simulink model "PTEngineCU"  (Simulink 10.1)
settings: Solver=ode45  StartTime=0.0  StopTime=inf  RelTol=1e-3  EnableMultiTasking=on
PreLoadFcn:
  | Trq_x = [500.0, 600.0, 700.0, 800.0, 1000.0, 2000.0, 3000.0, 4000.0, 4500.0, 5000.0, 6000.0, 7000.0, 8000.0];
  | TrqFull_y = [10.0, 40.0, 70.0, 95.0, 120.0, 145.0, 165.0, 180.0, 185.0, 182.0, 168.0, 130.0, 0.0];
  | 
  | TrqDrag_y = [-10.0, -10.0, -10.0, -10.0, -10.0, -20.0, -30.0, -40.0, -45.0, -50.0, -60.0, -70.0, -80.0];
  | 
  | TrqOpt_y = [0.0, 0.0, 0.0, 0.0, 0.0, 0.0, 0.0, 0.0, 0.0, 0.0, 0.0, 0.0, 0.0];
InitFcn:
  | Trq_x = [500.0, 600.0, 700.0, 800.0, 1000.0, 2000.0, 3000.0, 4000.0, 4500.0, 5000.0, 6000.0, 7000.0, 8000.0];
  | TrqFull_y = [10.0, 40.0, 70.0, 95.0, 120.0, 145.0, 165.0, 180.0, 185.0, 182.0, 168.0, 130.0, 0.0];
  | 
  | TrqDrag_y = [-10.0, -10.0, -10.0, -10.0, -10.0, -20.0, -30.0, -40.0, -45.0, -50.0, -60.0, -70.0, -80.0];
  | 
  | TrqOpt_y = [0.0, 0.0, 0.0, 0.0, 0.0, 0.0, 0.0, 0.0, 0.0, 0.0, 0.0, 0.0, 0.0];
libraries: simulink x7, CarMaker4SL x4
(part 2 of 2)

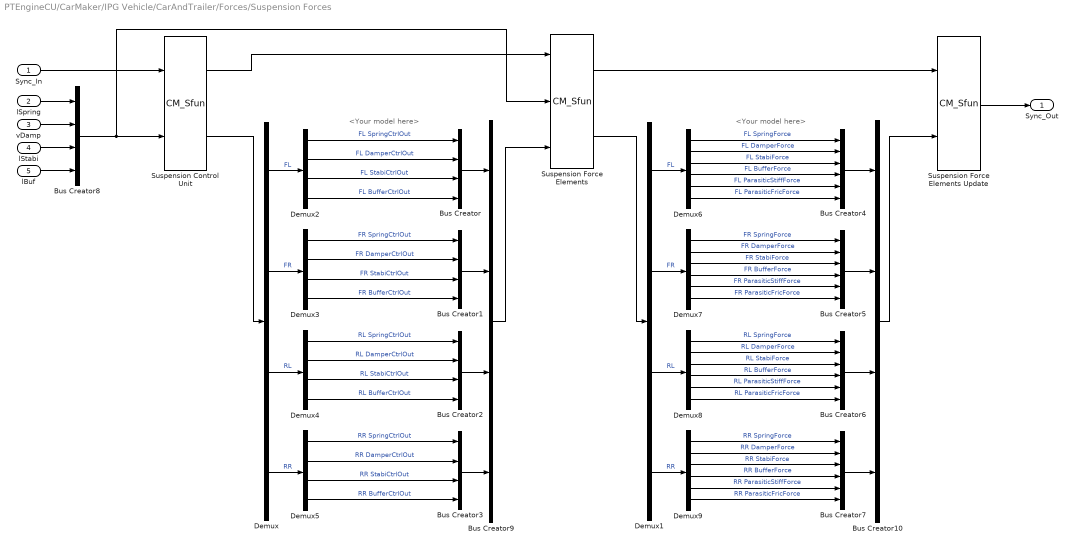
== system PTEngineCU/CarMaker/IPG Vehicle/CarAndTrailer/Forces/Suspension Forces ==
  note: <Your model here>
  note: <Your model here>
  Sync_In : Inport
  lSpring : Inport  Port=2
  vDamp : Inport  Port=3
  lStabi : Inport  Port=4
  lBuf : Inport  Port=5
  Bus Creator{,1..3,8..10} (7 alike) : BusCreator  Inputs=4
  Bus Creator{4..7} (4 alike) : BusCreator  Inputs=6
  Demux{,1..5} (6 alike) : Demux
  Demux{6..9} (4 alike) : Demux  Outputs=6
  Suspension Control Unit : S-Function  FunctionName=CM_Sfun  Parameters='ForcesSuspControl'  SFunctionDeploymentMode=off  EnableBusSupport=off
  Suspension Force Elements : S-Function  FunctionName=CM_Sfun  Parameters='ForcesSusp'  SFunctionDeploymentMode=off  EnableBusSupport=off
  Suspension Force Elements Update : S-Function  FunctionName=CM_Sfun  Parameters='ForcesSuspUpd'  SFunctionDeploymentMode=off  EnableBusSupport=off
  Sync_Out : Outport  VectorParamsAs1DForOutWhenUnconnected=off
  wires:
  vDamp/1 -> Bus Creator8/2
  lStabi/1 -> Bus Creator8/3
  lBuf/1 -> Bus Creator8/4
  lSpring/1 -> Bus Creator8/1
  Bus Creator8/1 -> Suspension Control Unit/2, Suspension Force Elements/2
  Sync_In/1 -> Suspension Control Unit/1
  Suspension Control Unit/1 -> Suspension Force Elements/1
  Suspension Force Elements/1 -> Suspension Force Elements Update/1
  Suspension Force Elements Update/1 -> Sync_Out/1
  Bus Creator4/1 -> Bus Creator10/1
  Bus Creator5/1 -> Bus Creator10/2
  Bus Creator6/1 -> Bus Creator10/3
  Bus Creator7/1 -> Bus Creator10/4
  Demux6/1 -> Bus Creator4/1  "FL SpringForce"
  Demux9/1 -> Bus Creator7/1  "RR SpringForce"
  Demux9/2 -> Bus Creator7/2  "RR DamperForce"
  Demux9/3 -> Bus Creator7/3  "RR StabiForce"
  Demux9/4 -> Bus Creator7/4  "RR BufferForce"
  Demux9/5 -> Bus Creator7/5  "RR ParasiticStiffForce"
  Demux9/6 -> Bus Creator7/6  "RR ParasiticFricForce"
  Demux8/1 -> Bus Creator6/1  "RL SpringForce"
  Demux8/2 -> Bus Creator6/2  "RL DamperForce"
  Demux8/4 -> Bus Creator6/4  "RL BufferForce"
  Demux8/5 -> Bus Creator6/5  "RL ParasiticStiffForce"
  Demux8/6 -> Bus Creator6/6  "RL ParasiticFricForce"
  Demux8/3 -> Bus Creator6/3  "RL StabiForce"
  Demux7/1 -> Bus Creator5/1  "FR SpringForce"
  Demux7/2 -> Bus Creator5/2  "FR DamperForce"
  Demux7/3 -> Bus Creator5/3  "FR StabiForce"
  Demux7/4 -> Bus Creator5/4  "FR BufferForce"
  Demux7/5 -> Bus Creator5/5  "FR ParasiticStiffForce"
  Demux7/6 -> Bus Creator5/6  "FR ParasiticFricForce"
  Demux6/2 -> Bus Creator4/2  "FL DamperForce"
  Demux6/3 -> Bus Creator4/3  "FL StabiForce"
  Demux6/4 -> Bus Creator4/4  "FL BufferForce"
  Demux6/5 -> Bus Creator4/5  "FL ParasiticStiffForce"
  Demux6/6 -> Bus Creator4/6  "FL ParasiticFricForce"
  Bus Creator10/1 -> Suspension Force Elements Update/2
  Demux/1 -> Demux2/1  "FL"
  Bus Creator1/1 -> Bus Creator9/2
  Demux/2 -> Demux3/1  "FR"
  Bus Creator2/1 -> Bus Creator9/3
  Demux/3 -> Demux4/1  "RL"
  Bus Creator3/1 -> Bus Creator9/4
  Demux2/1 -> Bus Creator/1  "FL SpringCtrlOut"
  Demux/4 -> Demux5/1  "RR"
  Demux5/1 -> Bus Creator3/1  "RR SpringCtrlOut"
  Demux5/2 -> Bus Creator3/2  "RR DamperCtrlOut"
  Demux5/3 -> Bus Creator3/3  "RR StabiCtrlOut"
  Demux5/4 -> Bus Creator3/4  "RR BufferCtrlOut"
  Demux4/1 -> Bus Creator2/1  "RL SpringCtrlOut"
  Demux4/2 -> Bus Creator2/2  "RL DamperCtrlOut"
  Demux4/4 -> Bus Creator2/4  "RL BufferCtrlOut"
  Demux4/3 -> Bus Creator2/3  "RL StabiCtrlOut"
  Demux3/1 -> Bus Creator1/1  "FR SpringCtrlOut"
  Demux3/2 -> Bus Creator1/2  "FR DamperCtrlOut"
  Demux3/3 -> Bus Creator1/3  "FR StabiCtrlOut"
  Demux3/4 -> Bus Creator1/4  "FR BufferCtrlOut"
  Demux2/2 -> Bus Creator/2  "FL DamperCtrlOut"
  Demux2/3 -> Bus Creator/3  "FL StabiCtrlOut"
  Demux2/4 -> Bus Creator/4  "FL BufferCtrlOut"
  Suspension Control Unit/2 -> Demux/1
  Bus Creator9/1 -> Suspension Force Elements/3
  Bus Creator/1 -> Bus Creator9/1
  Suspension Force Elements/2 -> Demux1/1
  Demux1/1 -> Demux6/1  "FL"
  Demux1/2 -> Demux7/1  "FR"
  Demux1/3 -> Demux8/1  "RL"
  Demux1/4 -> Demux9/1  "RR"

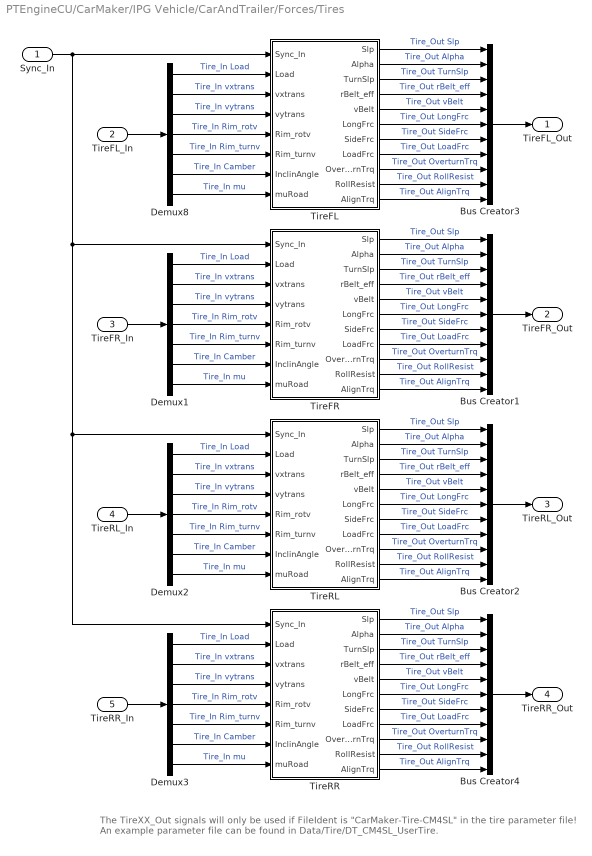
== system PTEngineCU/CarMaker/IPG Vehicle/CarAndTrailer/Forces/Tires ==
  note: The TireXX_Out signals will only be used if FileIdent is "CarMaker-Tire-CM4SL" in the tire parameter file!
      | An example parameter file can be found in Data/Tire/DT_CM4SL_UserTire.
  Sync_In : Inport
  TireFL_In : Inport  Port=2
  TireFR_In : Inport  Port=3
  TireRL_In : Inport  Port=4
  TireRR_In : Inport  Port=5
  Bus Creator{1..4} (4 alike) : BusCreator  Inputs=11
  Demux{1..3,8} (4 alike) : Demux  Outputs=7
      settings: DisplayOption=none
  TireFL : Subsystem
  TireFR : Subsystem
  TireRL : Subsystem
  TireRR : Subsystem
  TireFL_Out : Outport  VectorParamsAs1DForOutWhenUnconnected=off
  TireFR_Out : Outport  Port=2  VectorParamsAs1DForOutWhenUnconnected=off
  TireRL_Out : Outport  Port=3  VectorParamsAs1DForOutWhenUnconnected=off
  TireRR_Out : Outport  Port=4  VectorParamsAs1DForOutWhenUnconnected=off
  wires:
  Sync_In/1 -> TireRR/1(Sync_In), TireRL/1(Sync_In), TireFR/1(Sync_In), TireFL/1(Sync_In)
  Bus Creator4/1 -> TireRR_Out/1
  Bus Creator2/1 -> TireRL_Out/1
  Bus Creator1/1 -> TireFR_Out/1
  Demux3/5 -> TireRR/6(Rim_turnv)  "Tire_In Rim_turnv"
  Demux3/4 -> TireRR/5(Rim_rotv)  "Tire_In Rim_rotv"
  Demux3/1 -> TireRR/2(Load)  "Tire_In Load"
  Demux3/7 -> TireRR/8(muRoad)  "Tire_In mu"
  Demux3/6 -> TireRR/7(InclinAngle)  "Tire_In Camber"
  Demux3/2 -> TireRR/3(vxtrans)  "Tire_In vxtrans"
  Demux3/3 -> TireRR/4(vytrans)  "Tire_In vytrans"
  TireRR/11(AlignTrq) -> Bus Creator4/11  "Tire_Out AlignTrq"
  TireRR/10(RollResist) -> Bus Creator4/10  "Tire_Out RollResist"
  TireRR/9(OverturnTrq) -> Bus Creator4/9  "Tire_Out OverturnTrq"
  TireRR/8(LoadFrc) -> Bus Creator4/8  "Tire_Out LoadFrc"
  TireRR/7(SideFrc) -> Bus Creator4/7  "Tire_Out SideFrc"
  TireRR/6(LongFrc) -> Bus Creator4/6  "Tire_Out LongFrc"
  TireRR/5(vBelt) -> Bus Creator4/5  "Tire_Out vBelt"
  TireRR/4(rBelt_eff) -> Bus Creator4/4  "Tire_Out rBelt_eff"
  TireRR/3(TurnSlp) -> Bus Creator4/3  "Tire_Out TurnSlp"
  TireRR/1(Slp) -> Bus Creator4/1  "Tire_Out Slp"
  TireRR/2(Alpha) -> Bus Creator4/2  "Tire_Out Alpha"
  Demux2/5 -> TireRL/6(Rim_turnv)  "Tire_In Rim_turnv"
  Demux2/4 -> TireRL/5(Rim_rotv)  "Tire_In Rim_rotv"
  Demux2/1 -> TireRL/2(Load)  "Tire_In Load"
  Demux2/7 -> TireRL/8(muRoad)  "Tire_In mu"
  Demux2/6 -> TireRL/7(InclinAngle)  "Tire_In Camber"
  Demux2/2 -> TireRL/3(vxtrans)  "Tire_In vxtrans"
  Demux2/3 -> TireRL/4(vytrans)  "Tire_In vytrans"
  TireRL/11(AlignTrq) -> Bus Creator2/11  "Tire_Out AlignTrq"
  TireRL/10(RollResist) -> Bus Creator2/10  "Tire_Out RollResist"
  TireRL/9(OverturnTrq) -> Bus Creator2/9  "Tire_Out OverturnTrq"
  TireRL/8(LoadFrc) -> Bus Creator2/8  "Tire_Out LoadFrc"
  TireRL/7(SideFrc) -> Bus Creator2/7  "Tire_Out SideFrc"
  TireRL/6(LongFrc) -> Bus Creator2/6  "Tire_Out LongFrc"
  TireRL/5(vBelt) -> Bus Creator2/5  "Tire_Out vBelt"
  TireRL/4(rBelt_eff) -> Bus Creator2/4  "Tire_Out rBelt_eff"
  TireRL/3(TurnSlp) -> Bus Creator2/3  "Tire_Out TurnSlp"
  TireRL/1(Slp) -> Bus Creator2/1  "Tire_Out Slp"
  TireRL/2(Alpha) -> Bus Creator2/2  "Tire_Out Alpha"
  Demux1/5 -> TireFR/6(Rim_turnv)  "Tire_In Rim_turnv"
  Demux1/4 -> TireFR/5(Rim_rotv)  "Tire_In Rim_rotv"
  Demux1/1 -> TireFR/2(Load)  "Tire_In Load"
  Demux1/7 -> TireFR/8(muRoad)  "Tire_In mu"
  Demux1/6 -> TireFR/7(InclinAngle)  "Tire_In Camber"
  Demux1/2 -> TireFR/3(vxtrans)  "Tire_In vxtrans"
  Demux1/3 -> TireFR/4(vytrans)  "Tire_In vytrans"
  TireFR/11(AlignTrq) -> Bus Creator1/11  "Tire_Out AlignTrq"
  TireFR/10(RollResist) -> Bus Creator1/10  "Tire_Out RollResist"
  TireFR/9(OverturnTrq) -> Bus Creator1/9  "Tire_Out OverturnTrq"
  TireFR/8(LoadFrc) -> Bus Creator1/8  "Tire_Out LoadFrc"
  TireFR/7(SideFrc) -> Bus Creator1/7  "Tire_Out SideFrc"
  TireFR/6(LongFrc) -> Bus Creator1/6  "Tire_Out LongFrc"
  TireFR/5(vBelt) -> Bus Creator1/5  "Tire_Out vBelt"
  TireFR/4(rBelt_eff) -> Bus Creator1/4  "Tire_Out rBelt_eff"
  TireFR/3(TurnSlp) -> Bus Creator1/3  "Tire_Out TurnSlp"
  TireFR/1(Slp) -> Bus Creator1/1  "Tire_Out Slp"
  TireFR/2(Alpha) -> Bus Creator1/2  "Tire_Out Alpha"
  Demux8/5 -> TireFL/6(Rim_turnv)  "Tire_In Rim_turnv"
  Demux8/4 -> TireFL/5(Rim_rotv)  "Tire_In Rim_rotv"
  TireFL_In/1 -> Demux8/1
  Demux8/1 -> TireFL/2(Load)  "Tire_In Load"
  Demux8/7 -> TireFL/8(muRoad)  "Tire_In mu"
  Demux8/6 -> TireFL/7(InclinAngle)  "Tire_In Camber"
  Demux8/2 -> TireFL/3(vxtrans)  "Tire_In vxtrans"
  Demux8/3 -> TireFL/4(vytrans)  "Tire_In vytrans"
  TireFL/11(AlignTrq) -> Bus Creator3/11  "Tire_Out AlignTrq"
  TireFL/10(RollResist) -> Bus Creator3/10  "Tire_Out RollResist"
  TireFL/9(OverturnTrq) -> Bus Creator3/9  "Tire_Out OverturnTrq"
  TireFL/8(LoadFrc) -> Bus Creator3/8  "Tire_Out LoadFrc"
  TireFL/7(SideFrc) -> Bus Creator3/7  "Tire_Out SideFrc"
  TireFL/6(LongFrc) -> Bus Creator3/6  "Tire_Out LongFrc"
  TireFL/5(vBelt) -> Bus Creator3/5  "Tire_Out vBelt"
  TireFL/4(rBelt_eff) -> Bus Creator3/4  "Tire_Out rBelt_eff"
  TireFL/3(TurnSlp) -> Bus Creator3/3  "Tire_Out TurnSlp"
  TireFL/1(Slp) -> Bus Creator3/1  "Tire_Out Slp"
  TireFL/2(Alpha) -> Bus Creator3/2  "Tire_Out Alpha"
  Bus Creator3/1 -> TireFL_Out/1
  TireFR_In/1 -> Demux1/1
  TireRL_In/1 -> Demux2/1
  TireRR_In/1 -> Demux3/1

== system PTEngineCU/CarMaker/IPG Vehicle/CarAndTrailer/Forces/Vehicle Forces ==
  Sync_In : Inport
  Bus Creator1 : BusCreator  Inputs=12
  Bus Creator8 : BusCreator  Inputs=16
  BusCreator1 : BusCreator  Inputs=4
  BusCreator2 : BusCreator  Inputs=9
  Demux : Demux  Outputs=16
      settings: DisplayOption=none
  Demux1 : Demux  Outputs=12
      settings: DisplayOption=none
  Demux2 : Demux  Outputs=13
      settings: DisplayOption=none
  Forces : S-Function  FunctionName=CM_Sfun  Parameters='Forces'  SFunctionDeploymentMode=off  EnableBusSupport=off
  Terminator : Terminator
  Sync_Out : Outport  VectorParamsAs1DForOutWhenUnconnected=off
  Car.Virtual : Outport  Port=2  VectorParamsAs1DForOutWhenUnconnected=off
  Car.Aero : Outport  Port=3  VectorParamsAs1DForOutWhenUnconnected=off
  Car.Load : Outport  Port=4  VectorParamsAs1DForOutWhenUnconnected=off
  wires:
  BusCreator1/1 -> Terminator/1  "Aero IF (in)"
  Demux2/13 -> BusCreator2/9  "car Aero Trq_1 z"
  Demux2/12 -> BusCreator2/8  "car Aero Trq_1 y"
  Demux2/11 -> BusCreator2/7  "car Aero Trq_1 x"
  Demux2/10 -> BusCreator2/6  "car Aero Frc_1 z"
  Demux2/9 -> BusCreator2/5  "car Aero Frc_1 y"
  Demux2/8 -> BusCreator2/4  "car Aero Frc_1 x"
  Demux2/7 -> BusCreator2/3  "car Aero PoA_1 z"
  Demux2/6 -> BusCreator2/2  "car Aero PoA_1 y"
  Demux2/5 -> BusCreator2/1  "car Aero PoA_1 x"
  Demux2/4 -> BusCreator1/4  "car Aero tau_1"
  Demux2/3 -> BusCreator1/3  "car Aero ApproachVel_1 z"
  Demux2/2 -> BusCreator1/2  "car Aero ApproachVel_1 y"
  Demux2/1 -> BusCreator1/1  "car Aero ApproachVel_1 x"
  Demux/16 -> Bus Creator8/16  "Car Load_3 tz"
  Demux/15 -> Bus Creator8/15  "Car Load_3 ty"
  Demux/14 -> Bus Creator8/14  "Car Load_3 tx"
  Demux/13 -> Bus Creator8/13  "Car Load_3 mass"
  Demux1/12 -> Bus Creator1/12  "Car Virtual Trq_0 z"
  Demux1/11 -> Bus Creator1/11  "Car Virtual Trq_0 y"
  Demux1/10 -> Bus Creator1/10  "Car Virtual Trq_0 x"
  Demux1/9 -> Bus Creator1/9  "Car Virtual Trq_1 z"
  Demux1/8 -> Bus Creator1/8  "Car Virtual Trq_1 y"
  Demux1/7 -> Bus Creator1/7  "Car Virtual Trq_1 x"
  Demux1/6 -> Bus Creator1/6  "Car Virtual Frc_0 z"
  Demux1/5 -> Bus Creator1/5  "Car Virtual Frc_0 y"
  Demux1/4 -> Bus Creator1/4  "Car Virtual Frc_0 x"
  Sync_In/1 -> Forces/1
  Forces/1 -> Sync_Out/1
  BusCreator2/1 -> Car.Aero/1
  Demux1/1 -> Bus Creator1/1  "Car Virtual Frc_1 x"
  Demux1/2 -> Bus Creator1/2  "Car Virtual Frc_1 y"
  Demux1/3 -> Bus Creator1/3  "Car Virtual Frc_1 z"
  Forces/3 -> Demux2/1
  Forces/2 -> Demux1/1
  Bus Creator1/1 -> Car.Virtual/1
  Bus Creator8/1 -> Car.Load/1
  Demux/1 -> Bus Creator8/1  "Car Load_0 mass"
  Demux/2 -> Bus Creator8/2  "Car Load_0 tx"
  Demux/3 -> Bus Creator8/3  "Car Load_0 ty"
  Demux/4 -> Bus Creator8/4  "Car Load_0 tz"
  Demux/5 -> Bus Creator8/5  "Car Load_1 mass"
  Demux/6 -> Bus Creator8/6  "Car Load_1 tx"
  Demux/7 -> Bus Creator8/7  "Car Load_1 ty"
  Demux/8 -> Bus Creator8/8  "Car Load_1 tz"
  Demux/9 -> Bus Creator8/9  "Car Load_2 mass"
  Demux/10 -> Bus Creator8/10  "Car Load_2 tx"
  Demux/11 -> Bus Creator8/11  "Car Load_2 ty"
  Demux/12 -> Bus Creator8/12  "Car Load_2 tz"
  Forces/4 -> Demux/1

== system PTEngineCU/CarMaker/IPG Vehicle/CarAndTrailer/Trailer/CreateBus Car.Hitch.FrcTrq ==
  In1 : Inport
  Bus Creator7 : BusCreator  Inputs=6
  Demux7 : Demux  Outputs=6
      settings: DisplayOption=none
  Out1 : Outport  VectorParamsAs1DForOutWhenUnconnected=off
  wires:
  In1/1 -> Demux7/1
  Bus Creator7/1 -> Out1/1
  Demux7/6 -> Bus Creator7/6  "Car Hitch Trq2Car z"
  Demux7/5 -> Bus Creator7/5  "Car Hitch Trq2Car y"
  Demux7/4 -> Bus Creator7/4  "Car Hitch Trq2Car x"
  Demux7/3 -> Bus Creator7/3  "Car Hitch Frc2Car z"
  Demux7/2 -> Bus Creator7/2  "Car Hitch Frc2Car y"
  Demux7/1 -> Bus Creator7/1  "Car Hitch Frc2Car x"

== system PTEngineCU/CarMaker/IPG Vehicle/CarAndTrailer/Trailer/CreateBus Vhcl.Motion ==
  In1 : Inport
  BusCreator : BusCreator  Inputs=15
  Demux : Demux  Outputs=15
      settings: DisplayOption=none
  Out1 : Outport  VectorParamsAs1DForOutWhenUnconnected=off
  wires:
  Demux/15 -> BusCreator/15  "Vhcl YawAcc"
  Demux/14 -> BusCreator/14  "Vhcl YawVel"
  Demux/13 -> BusCreator/13  "Vhcl Yaw"
  Demux/12 -> BusCreator/12  "Vhcl PitchAcc"
  Demux/11 -> BusCreator/11  "Vhcl PitchVel"
  Demux/10 -> BusCreator/10  "Vhcl Pitch"
  Demux/9 -> BusCreator/9  "Vhcl RollAcc"
  Demux/8 -> BusCreator/8  "Vhcl RollVel"
  Demux/7 -> BusCreator/7  "Vhcl Roll"
  Demux/6 -> BusCreator/6  "Vhcl Hitch_Pos z"
  Demux/5 -> BusCreator/5  "Vhcl Hitch_Pos y"
  Demux/4 -> BusCreator/4  "Vhcl Hitch_Pos x"
  Demux/3 -> BusCreator/3  "Vhcl sRoad"
  Demux/2 -> BusCreator/2  "Vhcl Distance"
  Demux/1 -> BusCreator/1  "Vhcl v"
  In1/1 -> Demux/1
  BusCreator/1 -> Out1/1

== system PTEngineCU/CarMaker/IPG Vehicle/CarAndTrailer/Trailer/CreateBus Vhcl.PoI ==
  In1 : Inport
  Bus Creator3 : BusCreator  Inputs=18
  Demux3 : Demux  Outputs=18
      settings: DisplayOption=none
  Out1 : Outport  VectorParamsAs1DForOutWhenUnconnected=off
  wires:
  Demux3/18 -> Bus Creator3/18  "Vhcl PoI_GCS Elev"
  Demux3/17 -> Bus Creator3/17  "Vhcl PoI_GCS Lat"
  Demux3/16 -> Bus Creator3/16  "Vhcl PoI_GCS Long"
  Demux3/15 -> Bus Creator3/15  "Vhcl PoI_Acc_1 z"
  Demux3/14 -> Bus Creator3/14  "Vhcl PoI_Acc_1 y"
  Demux3/13 -> Bus Creator3/13  "Vhcl PoI_Acc_1 x"
  Demux3/12 -> Bus Creator3/12  "Vhcl PoI_Vel_1 z"
  Demux3/11 -> Bus Creator3/11  "Vhcl PoI_Vel_1 y"
  Demux3/10 -> Bus Creator3/10  "Vhcl PoI_Vel_1 x"
  Demux3/9 -> Bus Creator3/9  "Vhcl PoI_Acc z"
  Demux3/8 -> Bus Creator3/8  "Vhcl PoI_Acc y"
  Demux3/7 -> Bus Creator3/7  "Vhcl PoI_Acc x"
  Demux3/6 -> Bus Creator3/6  "Vhcl PoI_Vel z"
  Demux3/5 -> Bus Creator3/5  "Vhcl PoI_Vel y"
  Demux3/4 -> Bus Creator3/4  "Vhcl PoI_Vel x"
  Demux3/3 -> Bus Creator3/3  "Vhcl PoI_Pos z"
  Demux3/2 -> Bus Creator3/2  "Vhcl PoI_Pos y"
  In1/1 -> Demux3/1
  Bus Creator3/1 -> Out1/1
  Demux3/1 -> Bus Creator3/1  "Vhcl PoI_Pos x"

== system PTEngineCU/CarMaker/IPG Vehicle/CarAndTrailer/Trailer/CreateBus Vhcl.Steering ==
  In1 : Inport
  Bus Creator3 : BusCreator  Inputs=4
  Demux : Demux
      settings: DisplayOption=none
  Out1 : Outport  VectorParamsAs1DForOutWhenUnconnected=off
  wires:
  Bus Creator3/1 -> Out1/1
  Demux/1 -> Bus Creator3/1  "Vhcl Steering Ang"
  Demux/3 -> Bus Creator3/3  "Vhcl Steering AngAcc"
  Demux/2 -> Bus Creator3/2  "Vhcl Steering AngVel"
  Demux/4 -> Bus Creator3/4  "Vhcl Steering Trq"
  In1/1 -> Demux/1

== system PTEngineCU/CarMaker/IPG Vehicle/CarAndTrailer/Trailer/CreateBus Vhcl.Wheel.FL ==
  In1 : Inport
  Bus Creator3 : BusCreator  Inputs=14
  Demux3 : Demux  Outputs=14
      settings: DisplayOption=none
  Out1 : Outport  VectorParamsAs1DForOutWhenUnconnected=off
  wires:
  Demux3/14 -> Bus Creator3/14  "Vhcl Wheel FL Trq_WhlBearing"
  Demux3/13 -> Bus Creator3/13  "Vhcl Wheel FL Trq_T2W"
  Demux3/12 -> Bus Creator3/12  "Vhcl Wheel FL SideSlip"
  Demux3/11 -> Bus Creator3/11  "Vhcl Wheel FL LongSlip"
  Demux3/10 -> Bus Creator3/10  "Vhcl Wheel FL vBelt"
  Demux3/9 -> Bus Creator3/9  "Vhcl Wheel FL Fz"
  Demux3/8 -> Bus Creator3/8  "Vhcl Wheel FL Fy"
  Demux3/7 -> Bus Creator3/7  "Vhcl Wheel FL Fx"
  Demux3/6 -> Bus Creator3/6  "Vhcl Wheel FL r_zxy z"
  Demux3/5 -> Bus Creator3/5  "Vhcl Wheel FL r_zxy y"
  Demux3/4 -> Bus Creator3/4  "Vhcl Wheel FL r_zxy x"
  Demux3/3 -> Bus Creator3/3  "Vhcl Wheel FL t z"
  Demux3/2 -> Bus Creator3/2  "Vhcl Wheel FL t y"
  In1/1 -> Demux3/1
  Bus Creator3/1 -> Out1/1
  Demux3/1 -> Bus Creator3/1  "Vhcl Wheel FL t x"

== system PTEngineCU/CarMaker/IPG Vehicle/CarAndTrailer/Trailer/CreateBus Vhcl.Wheel.FR ==
  In1 : Inport
  Bus Creator3 : BusCreator  Inputs=14
  Demux3 : Demux  Outputs=14
      settings: DisplayOption=none
  Out1 : Outport  VectorParamsAs1DForOutWhenUnconnected=off
  wires:
  Demux3/14 -> Bus Creator3/14  "Vhcl Wheel FR Trq_WhlBearing"
  Demux3/13 -> Bus Creator3/13  "Vhcl Wheel FR Trq_T2W"
  Demux3/12 -> Bus Creator3/12  "Vhcl Wheel FR SideSlip"
  Demux3/11 -> Bus Creator3/11  "Vhcl Wheel FR LongSlip"
  Demux3/10 -> Bus Creator3/10  "Vhcl Wheel FR vBelt"
  Demux3/9 -> Bus Creator3/9  "Vhcl Wheel FR Fz"
  Demux3/8 -> Bus Creator3/8  "Vhcl Wheel FR Fy"
  Demux3/7 -> Bus Creator3/7  "Vhcl Wheel FR Fx"
  Demux3/6 -> Bus Creator3/6  "Vhcl Wheel FR r_zxy z"
  Demux3/5 -> Bus Creator3/5  "Vhcl Wheel FR r_zxy y"
  Demux3/4 -> Bus Creator3/4  "Vhcl Wheel FR r_zxy x"
  Demux3/3 -> Bus Creator3/3  "Vhcl Wheel FR t z"
  Demux3/2 -> Bus Creator3/2  "Vhcl Wheel FR t y"
  In1/1 -> Demux3/1
  Bus Creator3/1 -> Out1/1
  Demux3/1 -> Bus Creator3/1  "Vhcl Wheel FR t x"

== system PTEngineCU/CarMaker/IPG Vehicle/CarAndTrailer/Trailer/CreateBus Vhcl.Wheel.RL ==
  In1 : Inport
  Bus Creator3 : BusCreator  Inputs=14
  Demux3 : Demux  Outputs=14
      settings: DisplayOption=none
  Out1 : Outport  VectorParamsAs1DForOutWhenUnconnected=off
  wires:
  Demux3/14 -> Bus Creator3/14  "Vhcl Wheel RL Trq_WhlBearing"
  Demux3/13 -> Bus Creator3/13  "Vhcl Wheel RL Trq_T2W"
  Demux3/12 -> Bus Creator3/12  "Vhcl Wheel RL SideSlip"
  Demux3/11 -> Bus Creator3/11  "Vhcl Wheel RL LongSlip"
  Demux3/10 -> Bus Creator3/10  "Vhcl Wheel RL vBelt"
  Demux3/9 -> Bus Creator3/9  "Vhcl Wheel RL Fz"
  Demux3/8 -> Bus Creator3/8  "Vhcl Wheel RL Fy"
  Demux3/7 -> Bus Creator3/7  "Vhcl Wheel RL Fx"
  Demux3/6 -> Bus Creator3/6  "Vhcl Wheel RL r_zxy z"
  Demux3/5 -> Bus Creator3/5  "Vhcl Wheel RL r_zxy y"
  Demux3/4 -> Bus Creator3/4  "Vhcl Wheel RL r_zxy x"
  Demux3/3 -> Bus Creator3/3  "Vhcl Wheel RL t z"
  Demux3/2 -> Bus Creator3/2  "Vhcl Wheel RL t y"
  In1/1 -> Demux3/1
  Bus Creator3/1 -> Out1/1
  Demux3/1 -> Bus Creator3/1  "Vhcl Wheel RL t x"

== system PTEngineCU/CarMaker/IPG Vehicle/CarAndTrailer/Trailer/CreateBus Vhcl.Wheel.RR ==
  In1 : Inport
  Bus Creator3 : BusCreator  Inputs=14
  Demux3 : Demux  Outputs=14
      settings: DisplayOption=none
  Out1 : Outport  VectorParamsAs1DForOutWhenUnconnected=off
  wires:
  Demux3/14 -> Bus Creator3/14  "Vhcl Wheel RR Trq_WhlBearing"
  Demux3/13 -> Bus Creator3/13  "Vhcl Wheel RR Trq_T2W"
  Demux3/12 -> Bus Creator3/12  "Vhcl Wheel RR SideSlip"
  Demux3/11 -> Bus Creator3/11  "Vhcl Wheel RR LongSlip"
  Demux3/10 -> Bus Creator3/10  "Vhcl Wheel RR vBelt"
  Demux3/9 -> Bus Creator3/9  "Vhcl Wheel RR Fz"
  Demux3/8 -> Bus Creator3/8  "Vhcl Wheel RR Fy"
  Demux3/7 -> Bus Creator3/7  "Vhcl Wheel RR Fx"
  Demux3/6 -> Bus Creator3/6  "Vhcl Wheel RR r_zxy z"
  Demux3/5 -> Bus Creator3/5  "Vhcl Wheel RR r_zxy y"
  Demux3/4 -> Bus Creator3/4  "Vhcl Wheel RR r_zxy x"
  Demux3/3 -> Bus Creator3/3  "Vhcl Wheel RR t z"
  Demux3/2 -> Bus Creator3/2  "Vhcl Wheel RR t y"
  In1/1 -> Demux3/1
  Bus Creator3/1 -> Out1/1
  Demux3/1 -> Bus Creator3/1  "Vhcl Wheel RR t x"

== system PTEngineCU/CarMaker/IPG Vehicle/PowerTrain/ECU Example/CreateBus ECU_IF Output ==
  In : Inport
  BusCreator : BusCreator  Inputs=7
  Demux : Demux  Outputs=7
      settings: DisplayOption=none
  Out : Outport  VectorParamsAs1DForOutWhenUnconnected=off
  wires:
  Demux/7 -> BusCreator/7  "ECU_Out TrqOpt"
  Demux/6 -> BusCreator/6  "ECU_Out TrqFull"
  Demux/5 -> BusCreator/5  "ECU_Out TrqDrag"
  Demux/4 -> BusCreator/4  "ECU_Out Load"
  Demux/3 -> BusCreator/3  "ECU_Out Engine_on"
  Demux/2 -> BusCreator/2  "ECU_Out FuelCutOff"
  Demux/1 -> BusCreator/1  "ECU_Out Status"
  BusCreator/1 -> Out/1
  In/1 -> Demux/1

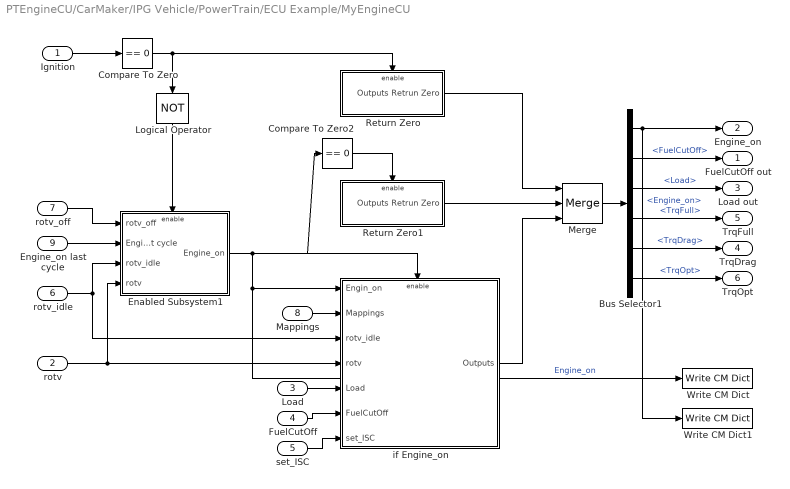
== system PTEngineCU/CarMaker/IPG Vehicle/PowerTrain/ECU Example/MyEngineCU ==
  Ignition : Inport
  rotv : Inport  Port=2
  Load : Inport  Port=3
  FuelCutOff : Inport  Port=4
  set_ISC : Inport  Port=5
  rotv_idle : Inport  Port=6
  rotv_off : Inport  Port=7
  Mappings : Inport  Port=8
  Engine_on last cycle : Inport  Port=9
  Bus Selector1 : BusSelector  OutputSignals=Engine_on,FuelCutOff,Load,TrqFull,TrqDrag,TrqOpt
  Compare To Zero : simulink/Logic and Bit Operations/Compare To Zero  relop===  OutDataTypeStr=uint8  ZeroCross=off
  Compare To Zero2 : simulink/Logic and Bit Operations/Compare To Zero  relop===  OutDataTypeStr=uint8  ZeroCross=off
  Enabled Subsystem1 : Subsystem  TreatAsAtomicUnit=on
  Logical Operator : Logic  Operator=NOT  AllPortsSameDT=off  OutDataTypeStr=boolean
  Merge : Merge  Inputs=3
  Return Zero : Subsystem  TreatAsAtomicUnit=on
  Return Zero1 : Subsystem  TreatAsAtomicUnit=on
  Write CM Dict : CarMaker4SL/Write CM Dict  xname=UserOut_00  xsync=off
  Write CM Dict1 : CarMaker4SL/Write CM Dict  xname=UserOut_01  xsync=off
  if Engine_on : Subsystem  TreatAsAtomicUnit=on
  FuelCutOff out : Outport  VectorParamsAs1DForOutWhenUnconnected=off
  Engine_on : Outport  Port=2  VectorParamsAs1DForOutWhenUnconnected=off
  Load out : Outport  Port=3  VectorParamsAs1DForOutWhenUnconnected=off
  TrqDrag : Outport  Port=4  VectorParamsAs1DForOutWhenUnconnected=off
  TrqFull : Outport  Port=5  VectorParamsAs1DForOutWhenUnconnected=off
  TrqOpt : Outport  Port=6  VectorParamsAs1DForOutWhenUnconnected=off
  wires:
  if Engine_on/1(Outputs) -> Merge/3
  Return Zero1/1(Outputs Retrun Zero) -> Merge/2
  Compare To Zero2/1 -> Return Zero1/Enable
  Bus Selector1/2 -> FuelCutOff out/1  "<FuelCutOff>"
  Bus Selector1/6 -> TrqOpt/1  "<TrqOpt>"
  Bus Selector1/4 -> TrqFull/1  "<TrqFull>"
  Bus Selector1/5 -> TrqDrag/1  "<TrqDrag>"
  Bus Selector1/3 -> Load out/1  "<Load>"
  Bus Selector1/1 -> Write CM Dict1/1, Engine_on/1  "<Engine_on>"
  Merge/1 -> Bus Selector1/1
  Return Zero/1(Outputs Retrun Zero) -> Merge/1
  set_ISC/1 -> if Engine_on/7(set_ISC)
  FuelCutOff/1 -> if Engine_on/6(FuelCutOff)
  Load/1 -> if Engine_on/5(Load)
  Engine_on last cycle/1 -> Enabled Subsystem1/2(Engine_on last cycle)
  rotv_off/1 -> Enabled Subsystem1/1(rotv_off)
  rotv_idle/1 -> if Engine_on/3(rotv_idle), Enabled Subsystem1/3(rotv_idle)
  rotv/1 -> if Engine_on/4(rotv), Enabled Subsystem1/4(rotv)
  Mappings/1 -> if Engine_on/2(Mappings)
  Enabled Subsystem1/1(Engine_on) -> Write CM Dict/1, if Engine_on/1(Engin_on), if Engine_on/Enable, Compare To Zero2/1  "Engine_on"
  Logical Operator/1 -> Enabled Subsystem1/Enable
  Compare To Zero/1 -> Return Zero/Enable, Logical Operator/1
  Ignition/1 -> Compare To Zero/1

== system PTEngineCU/CarMaker/IPG Vehicle/PowerTrain/ECU Example/PTEngineCU_In ==
  Sync_In : Inport
  CreateBus ECU_CfgIF : Subsystem
  CreateBus ECU_IF Input : Subsystem
  CreateBus PTEngineCU_In : BusCreator  Inputs=2
  S-Function : S-Function  FunctionName=cm_ptenginecu_in  SFunctionDeploymentMode=off  EnableBusSupport=off
  PTEngineCU_In : Outport  VectorParamsAs1DForOutWhenUnconnected=off
  wires:
  CreateBus ECU_IF Input/1(Out) -> CreateBus PTEngineCU_In/2  "ECU_IF Input"
  S-Function/2 -> CreateBus ECU_IF Input/1(In)
  CreateBus ECU_CfgIF/1(Out) -> CreateBus PTEngineCU_In/1  "ECU_CfgIF"
  S-Function/1 -> CreateBus ECU_CfgIF/1(In)
  CreateBus PTEngineCU_In/1 -> PTEngineCU_In/1
  Sync_In/1 -> S-Function/1

== system PTEngineCU/CarMaker/IPG Vehicle/PowerTrain/ECU Example/PTEngineCU_Out ==
  ECU_IF Output : Inport
  S-Function : S-Function  FunctionName=cm_ptenginecu_out  SFunctionDeploymentMode=off  EnableBusSupport=off
  wires:
  ECU_IF Output/1 -> S-Function/1

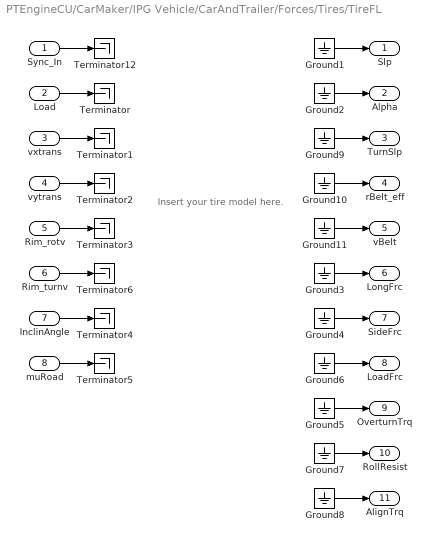
== system PTEngineCU/CarMaker/IPG Vehicle/CarAndTrailer/Forces/Tires/TireFL ==
  note: Insert your tire model here.
  Sync_In : Inport
  Load : Inport  Port=2
  vxtrans : Inport  Port=3
  vytrans : Inport  Port=4
  Rim_rotv : Inport  Port=5
  Rim_turnv : Inport  Port=6
  InclinAngle : Inport  Port=7
  muRoad : Inport  Port=8
  Ground{1..11} (11 alike) : Ground
  Terminator{,1..6,12} (8 alike) : Terminator
  Slp : Outport  VectorParamsAs1DForOutWhenUnconnected=off
  Alpha : Outport  Port=2  VectorParamsAs1DForOutWhenUnconnected=off
  TurnSlp : Outport  Port=3  VectorParamsAs1DForOutWhenUnconnected=off
  rBelt_eff : Outport  Port=4  VectorParamsAs1DForOutWhenUnconnected=off
  vBelt : Outport  Port=5  VectorParamsAs1DForOutWhenUnconnected=off
  LongFrc : Outport  Port=6  VectorParamsAs1DForOutWhenUnconnected=off
  SideFrc : Outport  Port=7  VectorParamsAs1DForOutWhenUnconnected=off
  LoadFrc : Outport  Port=8  VectorParamsAs1DForOutWhenUnconnected=off
  OverturnTrq : Outport  Port=9  VectorParamsAs1DForOutWhenUnconnected=off
  RollResist : Outport  Port=10  VectorParamsAs1DForOutWhenUnconnected=off
  AlignTrq : Outport  Port=11  VectorParamsAs1DForOutWhenUnconnected=off
  wires:
  Ground11/1 -> vBelt/1
  Ground10/1 -> rBelt_eff/1
  Ground9/1 -> TurnSlp/1
  Rim_turnv/1 -> Terminator6/1
  Sync_In/1 -> Terminator12/1
  Ground2/1 -> Alpha/1
  Ground3/1 -> LongFrc/1
  Ground4/1 -> SideFrc/1
  Ground5/1 -> OverturnTrq/1
  vxtrans/1 -> Terminator1/1
  vytrans/1 -> Terminator2/1
  Rim_rotv/1 -> Terminator3/1
  InclinAngle/1 -> Terminator4/1
  muRoad/1 -> Terminator5/1
  Load/1 -> Terminator/1
  Ground1/1 -> Slp/1
  Ground6/1 -> LoadFrc/1
  Ground7/1 -> RollResist/1
  Ground8/1 -> AlignTrq/1

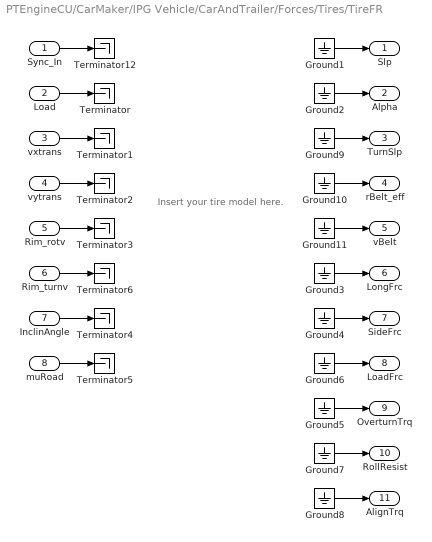
== system PTEngineCU/CarMaker/IPG Vehicle/CarAndTrailer/Forces/Tires/TireFR ==
  note: Insert your tire model here.
  Sync_In : Inport
  Load : Inport  Port=2
  vxtrans : Inport  Port=3
  vytrans : Inport  Port=4
  Rim_rotv : Inport  Port=5
  Rim_turnv : Inport  Port=6
  InclinAngle : Inport  Port=7
  muRoad : Inport  Port=8
  Ground{1..11} (11 alike) : Ground
  Terminator{,1..6,12} (8 alike) : Terminator
  Slp : Outport  VectorParamsAs1DForOutWhenUnconnected=off
  Alpha : Outport  Port=2  VectorParamsAs1DForOutWhenUnconnected=off
  TurnSlp : Outport  Port=3  VectorParamsAs1DForOutWhenUnconnected=off
  rBelt_eff : Outport  Port=4  VectorParamsAs1DForOutWhenUnconnected=off
  vBelt : Outport  Port=5  VectorParamsAs1DForOutWhenUnconnected=off
  LongFrc : Outport  Port=6  VectorParamsAs1DForOutWhenUnconnected=off
  SideFrc : Outport  Port=7  VectorParamsAs1DForOutWhenUnconnected=off
  LoadFrc : Outport  Port=8  VectorParamsAs1DForOutWhenUnconnected=off
  OverturnTrq : Outport  Port=9  VectorParamsAs1DForOutWhenUnconnected=off
  RollResist : Outport  Port=10  VectorParamsAs1DForOutWhenUnconnected=off
  AlignTrq : Outport  Port=11  VectorParamsAs1DForOutWhenUnconnected=off
  wires:
  Ground11/1 -> vBelt/1
  Ground10/1 -> rBelt_eff/1
  Ground9/1 -> TurnSlp/1
  Rim_turnv/1 -> Terminator6/1
  Sync_In/1 -> Terminator12/1
  Ground2/1 -> Alpha/1
  Ground3/1 -> LongFrc/1
  Ground4/1 -> SideFrc/1
  Ground5/1 -> OverturnTrq/1
  vxtrans/1 -> Terminator1/1
  vytrans/1 -> Terminator2/1
  Rim_rotv/1 -> Terminator3/1
  InclinAngle/1 -> Terminator4/1
  muRoad/1 -> Terminator5/1
  Load/1 -> Terminator/1
  Ground1/1 -> Slp/1
  Ground6/1 -> LoadFrc/1
  Ground7/1 -> RollResist/1
  Ground8/1 -> AlignTrq/1

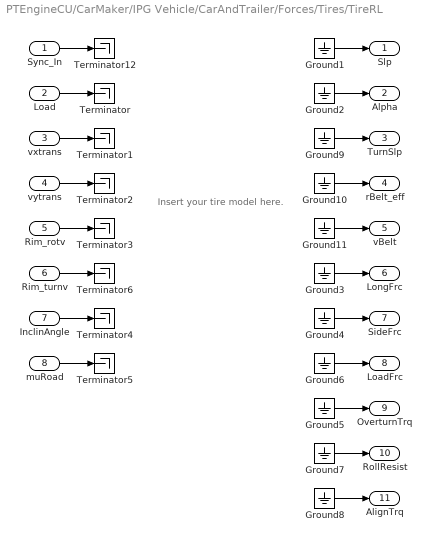
== system PTEngineCU/CarMaker/IPG Vehicle/CarAndTrailer/Forces/Tires/TireRL ==
  note: Insert your tire model here.
  Sync_In : Inport
  Load : Inport  Port=2
  vxtrans : Inport  Port=3
  vytrans : Inport  Port=4
  Rim_rotv : Inport  Port=5
  Rim_turnv : Inport  Port=6
  InclinAngle : Inport  Port=7
  muRoad : Inport  Port=8
  Ground{1..11} (11 alike) : Ground
  Terminator{,1..6,12} (8 alike) : Terminator
  Slp : Outport  VectorParamsAs1DForOutWhenUnconnected=off
  Alpha : Outport  Port=2  VectorParamsAs1DForOutWhenUnconnected=off
  TurnSlp : Outport  Port=3  VectorParamsAs1DForOutWhenUnconnected=off
  rBelt_eff : Outport  Port=4  VectorParamsAs1DForOutWhenUnconnected=off
  vBelt : Outport  Port=5  VectorParamsAs1DForOutWhenUnconnected=off
  LongFrc : Outport  Port=6  VectorParamsAs1DForOutWhenUnconnected=off
  SideFrc : Outport  Port=7  VectorParamsAs1DForOutWhenUnconnected=off
  LoadFrc : Outport  Port=8  VectorParamsAs1DForOutWhenUnconnected=off
  OverturnTrq : Outport  Port=9  VectorParamsAs1DForOutWhenUnconnected=off
  RollResist : Outport  Port=10  VectorParamsAs1DForOutWhenUnconnected=off
  AlignTrq : Outport  Port=11  VectorParamsAs1DForOutWhenUnconnected=off
  wires:
  Ground11/1 -> vBelt/1
  Ground10/1 -> rBelt_eff/1
  Ground9/1 -> TurnSlp/1
  Rim_turnv/1 -> Terminator6/1
  Sync_In/1 -> Terminator12/1
  Ground2/1 -> Alpha/1
  Ground3/1 -> LongFrc/1
  Ground4/1 -> SideFrc/1
  Ground5/1 -> OverturnTrq/1
  vxtrans/1 -> Terminator1/1
  vytrans/1 -> Terminator2/1
  Rim_rotv/1 -> Terminator3/1
  InclinAngle/1 -> Terminator4/1
  muRoad/1 -> Terminator5/1
  Load/1 -> Terminator/1
  Ground1/1 -> Slp/1
  Ground6/1 -> LoadFrc/1
  Ground7/1 -> RollResist/1
  Ground8/1 -> AlignTrq/1

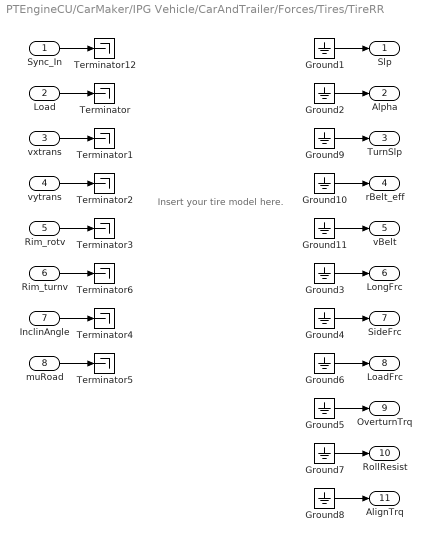
== system PTEngineCU/CarMaker/IPG Vehicle/CarAndTrailer/Forces/Tires/TireRR ==
  note: Insert your tire model here.
  Sync_In : Inport
  Load : Inport  Port=2
  vxtrans : Inport  Port=3
  vytrans : Inport  Port=4
  Rim_rotv : Inport  Port=5
  Rim_turnv : Inport  Port=6
  InclinAngle : Inport  Port=7
  muRoad : Inport  Port=8
  Ground{1..11} (11 alike) : Ground
  Terminator{,1..6,12} (8 alike) : Terminator
  Slp : Outport  VectorParamsAs1DForOutWhenUnconnected=off
  Alpha : Outport  Port=2  VectorParamsAs1DForOutWhenUnconnected=off
  TurnSlp : Outport  Port=3  VectorParamsAs1DForOutWhenUnconnected=off
  rBelt_eff : Outport  Port=4  VectorParamsAs1DForOutWhenUnconnected=off
  vBelt : Outport  Port=5  VectorParamsAs1DForOutWhenUnconnected=off
  LongFrc : Outport  Port=6  VectorParamsAs1DForOutWhenUnconnected=off
  SideFrc : Outport  Port=7  VectorParamsAs1DForOutWhenUnconnected=off
  LoadFrc : Outport  Port=8  VectorParamsAs1DForOutWhenUnconnected=off
  OverturnTrq : Outport  Port=9  VectorParamsAs1DForOutWhenUnconnected=off
  RollResist : Outport  Port=10  VectorParamsAs1DForOutWhenUnconnected=off
  AlignTrq : Outport  Port=11  VectorParamsAs1DForOutWhenUnconnected=off
  wires:
  Ground11/1 -> vBelt/1
  Ground10/1 -> rBelt_eff/1
  Ground9/1 -> TurnSlp/1
  Rim_turnv/1 -> Terminator6/1
  Sync_In/1 -> Terminator12/1
  Ground2/1 -> Alpha/1
  Ground3/1 -> LongFrc/1
  Ground4/1 -> SideFrc/1
  Ground5/1 -> OverturnTrq/1
  vxtrans/1 -> Terminator1/1
  vytrans/1 -> Terminator2/1
  Rim_rotv/1 -> Terminator3/1
  InclinAngle/1 -> Terminator4/1
  muRoad/1 -> Terminator5/1
  Load/1 -> Terminator/1
  Ground1/1 -> Slp/1
  Ground6/1 -> LoadFrc/1
  Ground7/1 -> RollResist/1
  Ground8/1 -> AlignTrq/1

== system PTEngineCU/CarMaker/IPG Vehicle/PowerTrain/ECU Example/MyEngineCU/Enabled Subsystem1 ==
  rotv_off : Inport
  Engine_on last cycle : Inport  Port=2
  rotv_idle : Inport  Port=3
  rotv : Inport  Port=4
  Enable : EnablePort
  Engine off : Subsystem  TreatAsAtomicUnit=on
  Engine on : Subsystem  TreatAsAtomicUnit=on
  Engine on? : If  NumInputs=3  IfExpression=u1 > u2  ElseIfExpressions=u1 < u3
  If Action Subsystem2 : Subsystem  TreatAsAtomicUnit=on
  Merge : Merge  Inputs=3
  Engine_on : Outport  VectorParamsAs1DForOutWhenUnconnected=off
  wires:
  Engine off/1(Engine_off) -> Merge/2
  Engine on/1(Engine_on) -> Merge/1
  If Action Subsystem2/1(Engine_on) -> Merge/3
  Merge/1 -> Engine_on/1
  Engine_on last cycle/1 -> If Action Subsystem2/1(Engine_on last cycle)
  Engine on?/3 -> If Action Subsystem2/Action
  Engine on?/2 -> Engine off/Action
  Engine on?/1 -> Engine on/Action
  rotv_off/1 -> Engine on?/3
  rotv_idle/1 -> Engine on?/2
  rotv/1 -> Engine on?/1

== system PTEngineCU/CarMaker/IPG Vehicle/PowerTrain/ECU Example/MyEngineCU/Return Zero ==
  Enable : EnablePort
  Bus Creator : BusCreator  Inputs=6
  Constant : Constant  Value=0
  Constant1 : Constant  Value=0
  Constant{2..5} (4 alike) : Constant  Value=0.0
  Outputs Retrun Zero : Outport  SampleTime=0.001  InitialOutput=0  VectorParamsAs1DForOutWhenUnconnected=off
  wires:
  Constant5/1 -> Bus Creator/6  "TrqOpt"
  Constant4/1 -> Bus Creator/5  "TrqDrag"
  Constant3/1 -> Bus Creator/4  "TrqFull"
  Constant2/1 -> Bus Creator/3  "Load"
  Constant1/1 -> Bus Creator/2  "FuelCutOff"
  Constant/1 -> Bus Creator/1  "Engine_on"
  Bus Creator/1 -> Outputs Retrun Zero/1

== system PTEngineCU/CarMaker/IPG Vehicle/PowerTrain/ECU Example/MyEngineCU/Return Zero1 ==
  Enable : EnablePort
  Bus Creator : BusCreator  Inputs=6
  Constant : Constant  Value=0
  Constant1 : Constant  Value=0
  Constant{2..5} (4 alike) : Constant  Value=0.0
  Outputs Retrun Zero : Outport  SampleTime=0.001  InitialOutput=0  VectorParamsAs1DForOutWhenUnconnected=off
  wires:
  Bus Creator/1 -> Outputs Retrun Zero/1
  Constant/1 -> Bus Creator/1  "Engine_on"
  Constant1/1 -> Bus Creator/2  "FuelCutOff"
  Constant2/1 -> Bus Creator/3  "Load"
  Constant3/1 -> Bus Creator/4  "TrqFull"
  Constant4/1 -> Bus Creator/5  "TrqDrag"
  Constant5/1 -> Bus Creator/6  "TrqOpt"

== system PTEngineCU/CarMaker/IPG Vehicle/PowerTrain/ECU Example/MyEngineCU/if Engine_on ==
  Engin_on : Inport
  Mappings : Inport  Port=2
  rotv_idle : Inport  Port=3
  rotv : Inport  Port=4
  Load : Inport  Port=5
  FuelCutOff : Inport  Port=6
  set_ISC : Inport  Port=7
  Enable : EnablePort
  == NOTSET : simulink/Logic and Bit Operations/Compare To Constant  relop===  const=-9999  OutDataTypeStr=uint8  ZeroCross=off
  Bus Creator : BusCreator  Inputs=6
  Bus Selector4 : BusSelector  OutputSignals=TrqFull,TrqDrag,TrqOpt
  Constant : Constant  Value=0.0
  FuelCutOff Function : Subsystem
  Gain : Gain
  Idle Speed Control : Subsystem
  Switch : Switch  Criteria=u2 ~= 0
  TrqFull & TrqDrag & TrqOpt : Subsystem
  Outputs : Outport  VectorParamsAs1DForOutWhenUnconnected=off
  wires:
  Gain/1 -> Bus Creator/1  "Engine_on"
  Bus Selector4/3 -> Bus Creator/6  "<TrqOpt>"
  Bus Selector4/2 -> Bus Creator/5  "<TrqDrag>"
  Bus Selector4/1 -> Bus Creator/4  "<TrqFull>"
  FuelCutOff Function/2(Load1) -> Bus Creator/3  "Load"
  FuelCutOff Function/1(FuelCutOff1) -> Bus Creator/2  "FuelCutOff"
  Engin_on/1 -> Gain/1
  Switch/1 -> Idle Speed Control/3(Load)  "Load"
  set_ISC/1 -> Idle Speed Control/2(set_ISC)
  rotv_idle/1 -> Idle Speed Control/1(rotv_idle)
  Idle Speed Control/1(Load_out) -> FuelCutOff Function/2(Load)
  FuelCutOff/1 -> FuelCutOff Function/1(FuelCutOff)
  TrqFull & TrqDrag & TrqOpt/1(Trg) -> Bus Selector4/1
  Constant/1 -> Switch/1
  == NOTSET/1 -> Switch/2
  Load/1 -> Switch/3, == NOTSET/1
  rotv/1 -> Idle Speed Control/4(rotv), FuelCutOff Function/3(rotv), TrqFull & TrqDrag & TrqOpt/1(rotv)
  Mappings/1 -> TrqFull & TrqDrag & TrqOpt/2(Mappings)
  Bus Creator/1 -> Outputs/1

== system PTEngineCU/CarMaker/IPG Vehicle/PowerTrain/ECU Example/PTEngineCU_In/CreateBus ECU_CfgIF ==
  In : Inport
  BusCreator : BusCreator  Inputs=4
  Demux : Demux
      settings: DisplayOption=none
  Out : Outport  VectorParamsAs1DForOutWhenUnconnected=off
  wires:
  Demux/4 -> BusCreator/4  "ECU_Cfg rotv_opt"
  Demux/3 -> BusCreator/3  "ECU_Cfg rotv_idle"
  Demux/2 -> BusCreator/2  "ECU_Cfg rotv_max"
  Demux/1 -> BusCreator/1  "ECU_Cfg rotv_off"
  BusCreator/1 -> Out/1
  In/1 -> Demux/1

== system PTEngineCU/CarMaker/IPG Vehicle/PowerTrain/ECU Example/PTEngineCU_In/CreateBus ECU_IF Input ==
  In : Inport
  BusCreator : BusCreator  Inputs=10
  Demux : Demux  Outputs=10
      settings: DisplayOption=none
  Out : Outport  VectorParamsAs1DForOutWhenUnconnected=off
  wires:
  Demux/10 -> BusCreator/10  "ECU FuelFlow"
  Demux/9 -> BusCreator/9  "ECU rot"
  Demux/8 -> BusCreator/8  "ECU rotv"
  Demux/7 -> BusCreator/7  "ECU rotv_trg"
  Demux/6 -> BusCreator/6  "ECU Trq"
  Demux/5 -> BusCreator/5  "ECU Trq_trg"
  Demux/4 -> BusCreator/4  "ECU Load"
  Demux/3 -> BusCreator/3  "ECU FuelCutOff"
  Demux/2 -> BusCreator/2  "ECU set_ISC"
  Demux/1 -> BusCreator/1  "ECU Ignition"
  BusCreator/1 -> Out/1
  In/1 -> Demux/1

== system PTEngineCU/CarMaker/IPG Vehicle/PowerTrain/ECU Example/MyEngineCU/Enabled Subsystem1/Engine off ==
  Action Port : ActionPort
  Constant : Constant  Value=0
  Engine_off : Outport  InitialOutput=0  VectorParamsAs1DForOutWhenUnconnected=off
  wires:
  Constant/1 -> Engine_off/1

== system PTEngineCU/CarMaker/IPG Vehicle/PowerTrain/ECU Example/MyEngineCU/Enabled Subsystem1/Engine on ==
  Action Port : ActionPort
  Constant : Constant
  Engine_on : Outport  InitialOutput=1  VectorParamsAs1DForOutWhenUnconnected=off
  wires:
  Constant/1 -> Engine_on/1

== system PTEngineCU/CarMaker/IPG Vehicle/PowerTrain/ECU Example/MyEngineCU/Enabled Subsystem1/If Action Subsystem2 ==
  Engine_on last cycle : Inport
  Action Port : ActionPort
  Engine_on : Outport  VectorParamsAs1DForOutWhenUnconnected=off
  wires:
  Engine_on last cycle/1 -> Engine_on/1

== system PTEngineCU/CarMaker/IPG Vehicle/PowerTrain/ECU Example/MyEngineCU/if Engine_on/FuelCutOff Function ==
  FuelCutOff : Inport
  Load : Inport  Port=2
  rotv : Inport  Port=3
  If : If  IfExpression=u1 == 1  ElseIfExpressions=u1 == -99999
  If Action Subsystem : Subsystem  TreatAsAtomicUnit=on
  If Action Subsystem1 : Subsystem  TreatAsAtomicUnit=on
  If Action Subsystem2 : Subsystem  TreatAsAtomicUnit=on
  Merge : Merge  Inputs=3
  Merge1 : Merge  Inputs=3
  Read CM Parameter : CarMaker4SL/Read CM Parameter  xfile=Vehicle  xkey=PowerTrain.ECU.FuelCutOff  xnout=1  xdefaults=1600  xmuxed=on
  rpm2radsec : Gain  Gain=0.104719755
  FuelCutOff1 : Outport  VectorParamsAs1DForOutWhenUnconnected=off
  Load1 : Outport  Port=2  VectorParamsAs1DForOutWhenUnconnected=off
  wires:
  rpm2radsec/1 -> If Action Subsystem2/3(nFuelCutOff)
  Load/1 -> If Action Subsystem2/1(Load), If Action Subsystem1/2(Load)  "Load"
  FuelCutOff/1 -> If Action Subsystem1/1(FuelCutOff), If Action Subsystem/1(FuelCutOff), If/1
  Merge1/1 -> Load1/1
  Merge/1 -> FuelCutOff1/1
  Read CM Parameter/1 -> rpm2radsec/1
  rotv/1 -> If Action Subsystem2/2(rotv)
  If Action Subsystem/2(Load out) -> Merge1/1
  If Action Subsystem1/2(Load out) -> Merge1/2
  If Action Subsystem2/2(Load out) -> Merge1/3
  If Action Subsystem2/1(FuelCutOff out) -> Merge/3
  If Action Subsystem1/1(FuelCutOff out) -> Merge/2
  If Action Subsystem/1(FuelCutOff out) -> Merge/1
  If/1 -> If Action Subsystem/Action
  If/2 -> If Action Subsystem2/Action
  If/3 -> If Action Subsystem1/Action

== system PTEngineCU/CarMaker/IPG Vehicle/PowerTrain/ECU Example/MyEngineCU/if Engine_on/Idle Speed Control ==
  rotv_idle : Inport
  set_ISC : Inport  Port=2
  Load : Inport  Port=3
  rotv : Inport  Port=4
  Bus Creator1 : BusCreator  Inputs=2
  Bus Creator2 : BusCreator  Inputs=2
  Bus Selector : BusSelector  OutputSignals=Load_I,Load
  Constant2 : Constant  Value=0.0
  Load Copy : InportShadow  Port=3
  Load Copy2 : InportShadow  Port=3
  Memory1 : Memory  InheritSampleTime=on
  PI : Subsystem
  Saturation : Saturate  UpperLimit=1  LowerLimit=0
  Subtract : Sum  Inputs=+-
  Switch1 : Switch  Criteria=u2 ~= 0
  Switch2 : Switch  Criteria=u2 ~= 0
  if condition : Subsystem
  Load_out : Outport  VectorParamsAs1DForOutWhenUnconnected=off
  wires:
  Load Copy2/1 -> Switch1/3
  Load Copy/1 -> Bus Creator1/2
  PI/2(Load out) -> Bus Creator2/2
  Subtract/1 -> PI/3(drotv)  "drotv"
  Memory1/1 -> PI/1(ISCtrl.Load_I)
  Bus Selector/1 -> Memory1/1  "<Load_I>"
  Bus Selector/2 -> Switch1/1  "<Load>"
  PI/1(ISCtrl.Load_I out) -> Bus Creator2/1
  rotv/1 -> Subtract/2, if condition/2(rotv)
  rotv_idle/1 -> Subtract/1, if condition/1(rotv_idle)
  Saturation/1 -> Load_out/1
  Constant2/1 -> Bus Creator1/1  "Load_I"
  if condition/1(Boolean) -> Switch2/2
  Bus Creator2/1 -> Switch2/1
  Bus Creator1/1 -> Switch2/3
  Switch2/1 -> Bus Selector/1
  set_ISC/1 -> Switch1/2
  Load/1 -> PI/2(Load)
  Switch1/1 -> Saturation/1

== system PTEngineCU/CarMaker/IPG Vehicle/PowerTrain/ECU Example/MyEngineCU/if Engine_on/TrqFull & TrqDrag & TrqOpt ==
  rotv : Inport
  Mappings : Inport  Port=2
  Bus Creator1 : BusCreator  Inputs=3
  Bus Selector : BusSelector  OutputSignals=TrqFull,TrqDrag,TrqOpt
  Bus Selector1 : BusSelector  OutputSignals=x,z
  Bus Selector2 : BusSelector  OutputSignals=x,z
  Bus Selector3 : BusSelector  OutputSignals=x,z
  Lookup Table Dynamic : simulink/Lookup Tables/Lookup Table Dynamic  LookUpMeth=Interpolation-Use End Values  OutDataTypeStr=float('double')  OutputDataTypeScalingMode=Specify via dialog  OutDataType=float('double')  OutScaling=2^-10  DoSatur=off
  Lookup Table Dynamic1 : simulink/Lookup Tables/Lookup Table Dynamic  LookUpMeth=Interpolation-Use End Values  OutDataTypeStr=float('double')  OutputDataTypeScalingMode=Specify via dialog  OutDataType=float('double')  OutScaling=2^-10  DoSatur=off
  Lookup Table Dynamic2 : simulink/Lookup Tables/Lookup Table Dynamic  LookUpMeth=Interpolation-Use End Values  OutDataTypeStr=float('double')  OutputDataTypeScalingMode=Specify via dialog  OutDataType=float('double')  OutScaling=2^-10  DoSatur=off
  Trg : Outport  VectorParamsAs1DForOutWhenUnconnected=off
  wires:
  Mappings/1 -> Bus Selector/1
  Bus Creator1/1 -> Trg/1
  rotv/1 -> Lookup Table Dynamic2/1, Lookup Table Dynamic1/1, Lookup Table Dynamic/1
  Lookup Table Dynamic2/1 -> Bus Creator1/3  "TrqOpt"
  Lookup Table Dynamic1/1 -> Bus Creator1/2  "TrqDrag"
  Lookup Table Dynamic/1 -> Bus Creator1/1  "TrqFull"
  Bus Selector3/2 -> Lookup Table Dynamic2/3  "<z>"
  Bus Selector3/1 -> Lookup Table Dynamic2/2  "<x>"
  Bus Selector2/1 -> Lookup Table Dynamic1/2  "<x>"
  Bus Selector2/2 -> Lookup Table Dynamic1/3  "<z>"
  Bus Selector/3 -> Bus Selector3/1  "<TrqOpt>"
  Bus Selector/2 -> Bus Selector2/1  "<TrqDrag>"
  Bus Selector/1 -> Bus Selector1/1  "<TrqFull>"
  Bus Selector1/2 -> Lookup Table Dynamic/3  "<z>"
  Bus Selector1/1 -> Lookup Table Dynamic/2  "<x>"

== system PTEngineCU/CarMaker/IPG Vehicle/PowerTrain/ECU Example/MyEngineCU/if Engine_on/FuelCutOff Function/If Action Subsystem ==
  FuelCutOff : Inport
  Action Port : ActionPort
  Constant : Constant  Value=0.0
  FuelCutOff out : Outport  VectorParamsAs1DForOutWhenUnconnected=off
  Load out : Outport  Port=2  InitialOutput=0  VectorParamsAs1DForOutWhenUnconnected=off
  wires:
  FuelCutOff/1 -> FuelCutOff out/1
  Constant/1 -> Load out/1

== system PTEngineCU/CarMaker/IPG Vehicle/PowerTrain/ECU Example/MyEngineCU/if Engine_on/FuelCutOff Function/If Action Subsystem1 ==
  FuelCutOff : Inport
  Load : Inport  Port=2
  Action Port : ActionPort
  FuelCutOff out : Outport  VectorParamsAs1DForOutWhenUnconnected=off
  Load out : Outport  Port=2  VectorParamsAs1DForOutWhenUnconnected=off
  wires:
  FuelCutOff/1 -> FuelCutOff out/1
  Load/1 -> Load out/1

== system PTEngineCU/CarMaker/IPG Vehicle/PowerTrain/ECU Example/MyEngineCU/if Engine_on/FuelCutOff Function/If Action Subsystem2 ==
  Load : Inport
  rotv : Inport  Port=2
  nFuelCutOff : Inport  Port=3
  Action Port : ActionPort
  Compare To Constant : simulink/Logic and Bit Operations/Compare To Constant  relop=<=  const=1e-3  OutDataTypeStr=uint8  ZeroCross=off
  Constant : Constant
  Constant1 : Constant  Value=0
  Gain : Gain
  Logical Operator : Logic  AllPortsSameDT=off  OutDataTypeStr=boolean
  Relational Operator : RelationalOperator  OutDataTypeStr=boolean  RndMeth=Nearest
  Switch : Switch  Criteria=u2 ~= 0
  FuelCutOff out : Outport  VectorParamsAs1DForOutWhenUnconnected=off
  Load out : Outport  Port=2  VectorParamsAs1DForOutWhenUnconnected=off
  wires:
  Gain/1 -> Load out/1
  Constant1/1 -> Switch/3
  Constant/1 -> Switch/1
  Logical Operator/1 -> Switch/2
  Compare To Constant/1 -> Logical Operator/1
  Relational Operator/1 -> Logical Operator/2
  nFuelCutOff/1 -> Relational Operator/2
  rotv/1 -> Relational Operator/1
  Switch/1 -> FuelCutOff out/1
  Load/1 -> Gain/1, Compare To Constant/1

== system PTEngineCU/CarMaker/IPG Vehicle/PowerTrain/ECU Example/MyEngineCU/if Engine_on/Idle Speed Control/PI ==
  ISCtrl.Load_I : Inport
  Load : Inport  Port=2
  drotv : Inport  Port=3
  Add : Sum
  Add1 : Sum
  Constant : Constant  Value=0.0
  If : If  IfExpression=u1 < 1e-3
  If Action Subsystem : Subsystem  TreatAsAtomicUnit=on
  If Action Subsystem1 : Subsystem  TreatAsAtomicUnit=on
  Load1 : InportShadow  Port=2
  Max : MinMax  Function=max  Inputs=2
  Merge : Merge
  Merge1 : Merge
  Product : Product  RndMeth=Zero
  Read CM Parameter : CarMaker4SL/Read CM Parameter  xfile=Vehicle  xkey=PowerTrain.MyEngineCU.ISCtrl.P  xnout=1  xdefaults=0.1  xmuxed=on
  Saturation : Saturate  UpperLimit=1  LowerLimit=0
  ISCtrl.Load_I out : Outport  VectorParamsAs1DForOutWhenUnconnected=off
  Load out : Outport  Port=2  VectorParamsAs1DForOutWhenUnconnected=off
  wires:
  Saturation/1 -> Add/2
  Load1/1 -> If/1
  Merge1/1 -> ISCtrl.Load_I out/1  "Load_I"
  If Action Subsystem1/1(ISCtrl.Load_I out) -> Merge1/1
  If Action Subsystem1/2(Load_I out) -> Merge/1
  If/1 -> If Action Subsystem1/Action
  If Action Subsystem/1(ISCtrl.Load_I out) -> Merge1/2
  If Action Subsystem/2(Load_I out) -> Merge/2
  Merge/1 -> Add1/1
  If/2 -> If Action Subsystem/Action
  ISCtrl.Load_I/1 -> If Action Subsystem1/1(ISCtrl.Load_I), If Action Subsystem/1(ISCtrl.Load_I)
  Load/1 -> Add/1
  Constant/1 -> Max/2
  Max/1 -> Add1/2
  Product/1 -> Max/1
  Read CM Parameter/1 -> Product/2
  drotv/1 -> If Action Subsystem1/2(drotv), If Action Subsystem/2(drotv), Product/1
  Add1/1 -> Saturation/1
  Add/1 -> Load out/1  "Load"

== system PTEngineCU/CarMaker/IPG Vehicle/PowerTrain/ECU Example/MyEngineCU/if Engine_on/Idle Speed Control/if condition ==
  rotv_idle : Inport
  rotv : Inport  Port=2
  Add : Sum
  Constant1 : Constant  Value=200.0
  Relational Operator : RelationalOperator  Operator=<  OutDataTypeStr=boolean  RndMeth=Nearest
  rpm2radsec : Gain  Gain=0.104719755
  Boolean : Outport  VectorParamsAs1DForOutWhenUnconnected=off
  wires:
  Add/1 -> Relational Operator/2
  rotv/1 -> Relational Operator/1
  Relational Operator/1 -> Boolean/1
  rotv_idle/1 -> Add/1
  Constant1/1 -> rpm2radsec/1
  rpm2radsec/1 -> Add/2

== system PTEngineCU/CarMaker/IPG Vehicle/PowerTrain/ECU Example/MyEngineCU/if Engine_on/Idle Speed Control/PI/If Action Subsystem ==
  ISCtrl.Load_I : Inport
  drotv : Inport  Port=2
  Action Port : ActionPort
  Add : Sum
  Constant : Constant
  Constant1 : Constant  Value=200.0
  Divide : Product  Inputs=*/
  Gain : Gain
  Product : Product  RndMeth=Zero
  Saturation : Saturate  UpperLimit=1  LowerLimit=0
  rpm2radsec : Gain  Gain=0.104719755
  ISCtrl.Load_I out : Outport  VectorParamsAs1DForOutWhenUnconnected=off
  Load_I out : Outport  Port=2  VectorParamsAs1DForOutWhenUnconnected=off
  wires:
  Gain/1 -> ISCtrl.Load_I out/1
  Saturation/1 -> Product/2
  Constant1/1 -> rpm2radsec/1
  rpm2radsec/1 -> Divide/2
  drotv/1 -> Divide/1
  Divide/1 -> Add/2
  Constant/1 -> Add/1
  Add/1 -> Saturation/1  "fac"
  Product/1 -> Load_I out/1
  ISCtrl.Load_I/1 -> Gain/1, Product/1

== system PTEngineCU/CarMaker/IPG Vehicle/PowerTrain/ECU Example/MyEngineCU/if Engine_on/Idle Speed Control/PI/If Action Subsystem1 ==
  ISCtrl.Load_I : Inport
  drotv : Inport  Port=2
  Action Port : ActionPort
  Add : Sum
  Gain : Gain
  Gain1 : Gain
  ISCtrl_I : Constant  Value=0.01
  Product : Product  RndMeth=Zero
  Saturation : Saturate  UpperLimit=1  LowerLimit=0
  ISCtrl.Load_I out : Outport  VectorParamsAs1DForOutWhenUnconnected=off
  Load_I out : Outport  Port=2  VectorParamsAs1DForOutWhenUnconnected=off
  wires:
  Gain1/1 -> Load_I out/1
  Gain/1 -> ISCtrl.Load_I out/1
  ISCtrl_I/1 -> Product/2
  drotv/1 -> Product/1
  Product/1 -> Add/1
  ISCtrl.Load_I/1 -> Add/2
  Saturation/1 -> Gain1/1, Gain/1
  Add/1 -> Saturation/1
